simulink model "Long_sim"  (R2023a)
settings: Solver=VariableStepAuto  StartTime=0.0  StopTime=10.0  RelTol=1e-3
values from neighbouring files (symbols this model uses):
  A_FL = [Xu, Xw, -w0, -g*cos(theta0) ... (first row only)    [Approximations.m]
  B_FL = [Xde, Xdth ... (first row only)    [Approximations.m]
  C_FL = eye(4)    [Approximations.m]
  D_FL = zeros(4,2)    [Approximations.m]
undefined symbols (not defined in the file or in its folder): d_pitch, theta0, U0, w0, z0
libraries: simulink_extras x7, cstblocks x2
settings Model: Creator=podyd  LastModifiedBy=podyd

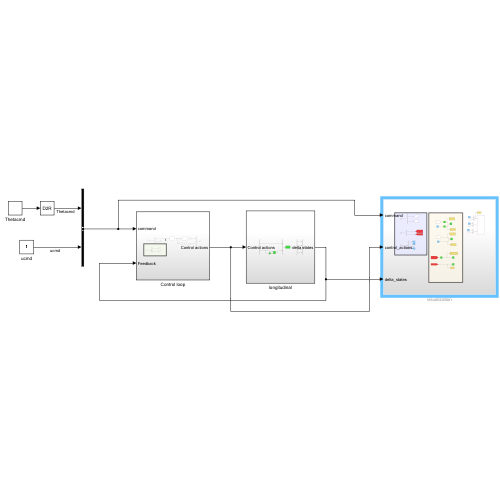
[thumbnail: Simulink's stored preview of the top-level diagram]
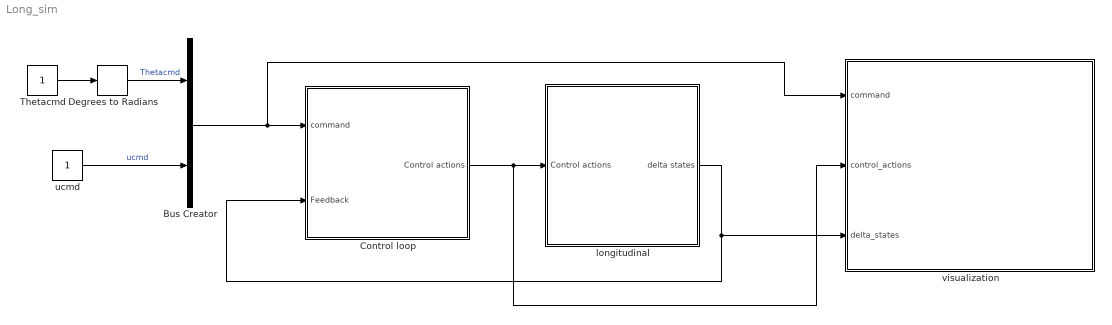
== system Long_sim ==
  Bus Creator : BusCreator  Inputs=2
  Control loop : Subsystem
  Degrees to Radians : simulink_extras/Transformations/Degrees to Radians
  Thetacmd : Constant
  longitudinal : Subsystem
  ucmd : Constant
  visualization : Subsystem
  wires:
  ucmd/1 -> Bus Creator/2  "ucmd"
  Thetacmd/1 -> Degrees to Radians/1
  Degrees to Radians/1 -> Bus Creator/1  "Thetacmd"
  Bus Creator/1 -> visualization/1(command), Control loop/1(command)
  longitudinal/1(delta states) -> visualization/3(delta_states), Control loop/2(Feedback)
  Control loop/1(Control actions) -> visualization/2(control_actions), longitudinal/1(Control actions)

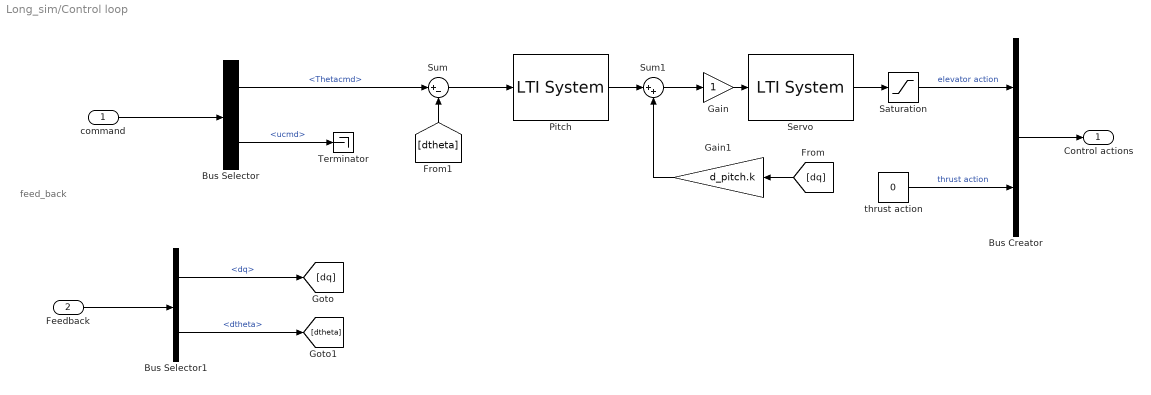
== system Long_sim/Control loop ==
  note: feed_back
  command : Inport
  Feedback : Inport  Port=2
  Bus Creator : BusCreator  Inputs=2
  Bus Selector : BusSelector  OutputSignals=Thetacmd,ucmd
  Bus Selector1 : BusSelector  OutputSignals=dq,dtheta
  Gain : Gain
  Gain1 : Gain  Gain=d_pitch.k
  Pitch : cstblocks/LTI System  sys=tf(1,[1 1])  IC=[]
  Saturation : Saturate
  Servo : cstblocks/LTI System  sys=servo  IC=[]
  Sum : Sum  Inputs=|+-
  Sum1 : Sum  Inputs=|++
  Terminator : Terminator
  thrust action : Constant  Value=0
  Control actions : Outport
  wires:
  command/1 -> Bus Selector/1
  Bus Selector/1 -> Sum/1  "<Thetacmd>"
  Bus Selector/2 -> Terminator/1  "<ucmd>"
  [dtheta] -> Sum/2
  Feedback/1 -> Bus Selector1/1
  Bus Selector1/1 -> [dq]  "<dq>"
  Bus Selector1/2 -> [dtheta]  "<dtheta>"
  Sum/1 -> Pitch/1
  Pitch/1 -> Sum1/1
  Sum1/1 -> Gain/1
  Gain/1 -> Servo/1
  Servo/1 -> Saturation/1
  [dq] -> Gain1/1
  Gain1/1 -> Sum1/2
  Saturation/1 -> Bus Creator/1  "elevator action"
  Bus Creator/1 -> Control actions/1
  thrust action/1 -> Bus Creator/2  "thrust action"

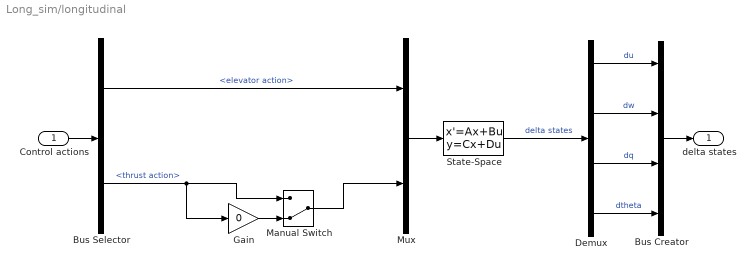
== system Long_sim/longitudinal ==
  Control actions : Inport
  Bus Creator : BusCreator  Inputs=4
  Bus Selector : BusSelector  OutputSignals=elevator action,thrust action
  Demux : Demux
  Gain : Gain  Gain=0
  Manual Switch : ManualSwitch  CurrentSetting=0
  Mux : Mux  Inputs=2
  State-Space : StateSpace  A=A_FL  B=B_FL  C=C_FL  D=D_FL  InitialCondition=0  ParameterTunability=Unconstrained
  delta states : Outport
  wires:
  Demux/4 -> Bus Creator/4  "dtheta"
  Bus Creator/1 -> delta states/1
  Manual Switch/1 -> Mux/2
  Mux/1 -> State-Space/1
  Demux/1 -> Bus Creator/1  "du"
  Demux/3 -> Bus Creator/3  "dq"
  Control actions/1 -> Bus Selector/1
  Demux/2 -> Bus Creator/2  "dw"
  Bus Selector/2 -> Gain/1, Manual Switch/1  "<thrust action>"
  Gain/1 -> Manual Switch/2
  State-Space/1 -> Demux/1  "delta states"
  Bus Selector/1 -> Mux/1  "<elevator action>"

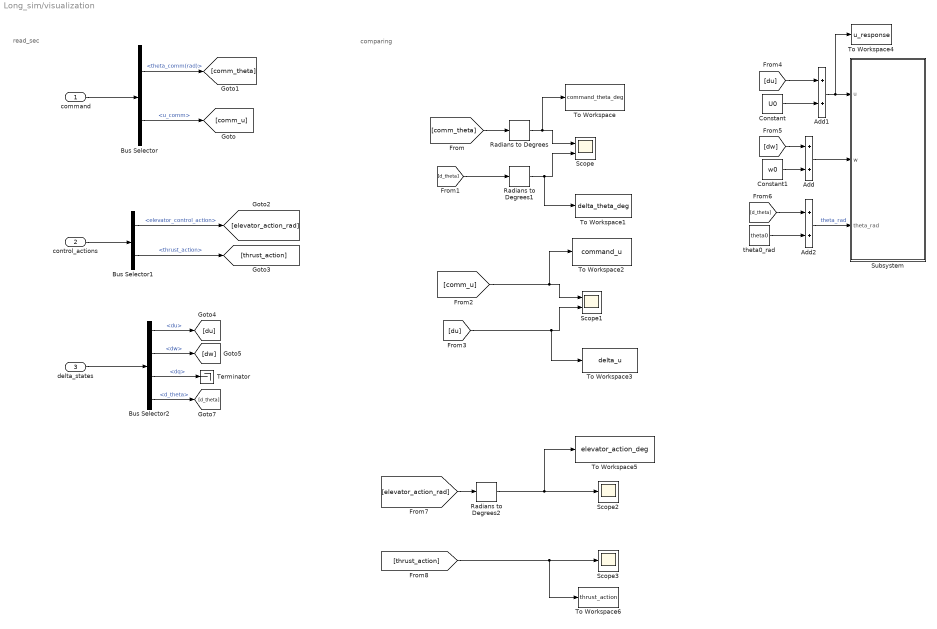
== system Long_sim/visualization ==
  note: comparing
  note: read_sec
  command : Inport
  control_actions : Inport  Port=2
  delta_states : Inport  Port=3
  Add : Sum
  Add1 : Sum
  Add2 : Sum
  Bus Selector : BusSelector  OutputSignals=theta_comm(rad),u_comm
  Bus Selector1 : BusSelector  OutputSignals=elevator_control_action,thrust_action
  Bus Selector2 : BusSelector  OutputSignals=du,dw,dq,d_theta
  Constant : Constant  Value=U0
  Constant1 : Constant  Value=w0
  Radians to Degrees : simulink_extras/Transformations/Radians to Degrees
  Radians to Degrees1 : simulink_extras/Transformations/Radians to Degrees
  Radians to Degrees2 : simulink_extras/Transformations/Radians to Degrees
  Scope : Scope  NumInputPorts=2
  Scope1 : Scope  NumInputPorts=2
  Scope2 : Scope
  Scope3 : Scope
  Subsystem : Subsystem
  Terminator : Terminator
  To Workspace : ToWorkspace  VariableName=command_theta_deg  SampleTime=-1
  To Workspace1 : ToWorkspace  VariableName=delta_theta_deg  SampleTime=-1
  To Workspace2 : ToWorkspace  VariableName=command_u  SampleTime=-1
  To Workspace3 : ToWorkspace  VariableName=delta_u  SampleTime=-1
  To Workspace4 : ToWorkspace  VariableName=u_response  SaveFormat=Timeseries  SampleTime=-1
  To Workspace5 : ToWorkspace  VariableName=elevator_action_deg  SampleTime=-1
  To Workspace6 : ToWorkspace  VariableName=thrust_action  SampleTime=-1
  theta0_rad : Constant  Value=theta0
  wires:
  command/1 -> Bus Selector/1
  control_actions/1 -> Bus Selector1/1
  delta_states/1 -> Bus Selector2/1
  Bus Selector/2 -> [comm_u]  "<u_comm>"
  Bus Selector/1 -> [comm_theta]  "<theta_comm(rad)>"
  Bus Selector1/1 -> [elevator_action_rad]  "<elevator_control_action>"
  Bus Selector1/2 -> [thrust_action]  "<thrust_action>"
  Bus Selector2/1 -> [du]  "<du>"
  Bus Selector2/3 -> Terminator/1  "<dq>"
  Bus Selector2/2 -> [dw]  "<dw>"
  Bus Selector2/4 -> [d_theta]  "<d_theta>"
  [comm_theta] -> Radians to Degrees/1
  [d_theta] -> Radians to Degrees1/1
  Radians to Degrees/1 -> To Workspace/1, Scope/1
  Radians to Degrees1/1 -> To Workspace1/1, Scope/2
  [comm_u] -> To Workspace2/1, Scope1/1
  [du] -> To Workspace3/1, Scope1/2
  [du] -> Add1/1
  Constant/1 -> Add1/2
  [dw] -> Add/1
  Constant1/1 -> Add/2
  [d_theta] -> Add2/1
  theta0_rad/1 -> Add2/2
  Add2/1 -> Subsystem/3(theta_rad)  "theta_rad"
  Add/1 -> Subsystem/2(w)
  Add1/1 -> To Workspace4/1, Subsystem/1(u)
  [elevator_action_rad] -> Radians to Degrees2/1
  [thrust_action] -> To Workspace6/1, Scope3/1
  Radians to Degrees2/1 -> To Workspace5/1, Scope2/1

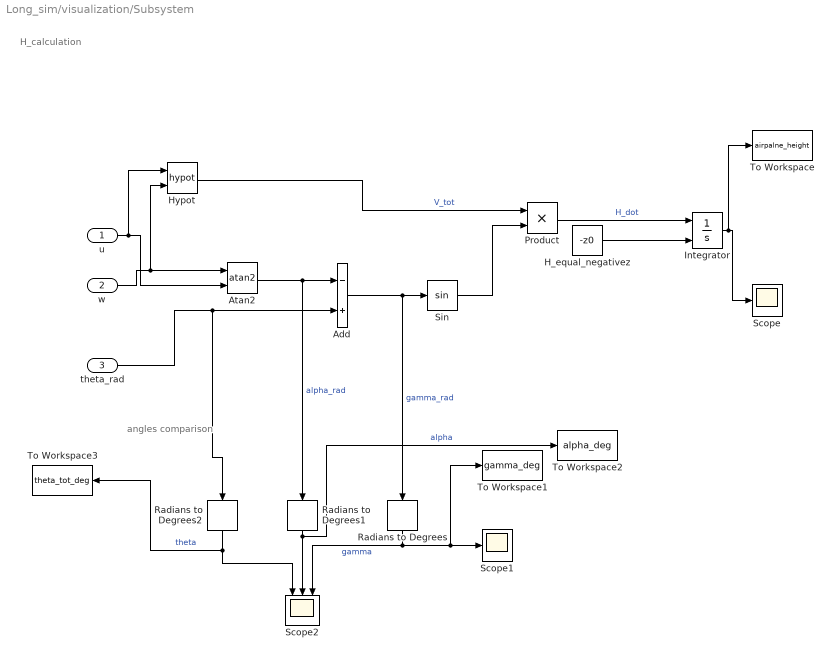
== system Long_sim/visualization/Subsystem ==
  note: angles comparison
  note: H_calculation
  u : Inport
  w : Inport  Port=2
  theta_rad : Inport  Port=3
  Add : Sum  Inputs=-+
  Atan2 : Trigonometry  Operator=atan2
  H_equal_negativez : Constant  Value=-z0
  Hypot : Math  Operator=hypot  SignedPower=on
  Integrator : Integrator  InitialConditionSource=external
  Product : Product
  Radians to Degrees : simulink_extras/Transformations/Radians to Degrees
  Radians to Degrees1 : simulink_extras/Transformations/Radians to Degrees
  Radians to Degrees2 : simulink_extras/Transformations/Radians to Degrees
  Scope : Scope
  Scope1 : Scope
  Scope2 : Scope  NumInputPorts=3
  Sin : Trigonometry
  To Workspace : ToWorkspace  VariableName=airpalne_height  SampleTime=-1
  To Workspace1 : ToWorkspace  VariableName=gamma_deg  SampleTime=-1
  To Workspace2 : ToWorkspace  VariableName=alpha_deg  SampleTime=-1
  To Workspace3 : ToWorkspace  VariableName=theta_tot_deg  SampleTime=-1
  wires:
  Atan2/1 -> Add/1, Radians to Degrees1/1  "alpha_rad"
  w/1 -> Hypot/2, Atan2/1
  u/1 -> Hypot/1, Atan2/2
  theta_rad/1 -> Add/2, Radians to Degrees2/1
  Add/1 -> Radians to Degrees/1, Sin/1  "gamma_rad"
  Hypot/1 -> Product/1  "V_tot"
  Sin/1 -> Product/2
  Product/1 -> Integrator/1  "H_dot"
  H_equal_negativez/1 -> Integrator/2
  Integrator/1 -> To Workspace/1, Scope/1
  Radians to Degrees/1 -> Scope2/3, To Workspace1/1, Scope1/1  "gamma"
  Radians to Degrees1/1 -> To Workspace2/1, Scope2/2  "alpha"
  Radians to Degrees2/1 -> To Workspace3/1, Scope2/1  "theta"
